simulink model "Quadcopter_Model_Linear"  (R2022a)
settings: Solver=ode45  StartTime=0.0  StopTime=20  RelTol=1e-3
values from neighbouring files (symbols this model uses):
  A = double(subs(a,[x_vec;u],equil))    [A_and_B_Matricies.m]    (also in Controller_LQR.m; Create_System.m; Linear_Main.mat = [0 0 0 0 0 0 0 0 0 0 0 0 ... (81 elements, 9x9)]; Linear_Model.mat = [0 0 0 0 0 0 0 0 0 0 0 1 ... (81 elements, 9x9)])
  B = double(subs(b,[x_vec;u],equil))    [A_and_B_Matricies.m]    (also in Controller_LQR.m; Create_System.m; Linear_Main.mat = [0 0 -1 0 13.2591958939 78.431372549 0 0 0 0 0 -1 ... (36 el; Linear_Model.mat = [0 13.2591958939 0 0 0 0 78.431372549 0 -1 0 0 0 ... (36 ele)
  u_e = zeros(4,1)    [A_and_B_Matricies.m]    (also in Controller_LQR.m; Create_System.m; Linear_Main.mat = [2.45 2.45 2.45 2.45]; Linear_Model.mat = [2.45 2.45 2.45 2.45])
undefined symbols (not defined in the file or in its folder): init, K1, K2, K3, K4
settings Model: Creator=vicen  LastModifiedBy=vicen
settings DebuggingCC: UnconnectedInputMsg=warning  UnconnectedOutputMsg=warning  UnconnectedLineMsg=warning
settings RTWCC: DLArmComputeVersion=19.05

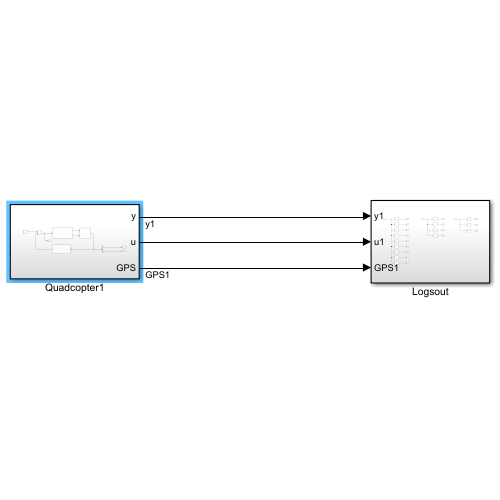
[thumbnail: Simulink's stored preview of the top-level diagram]
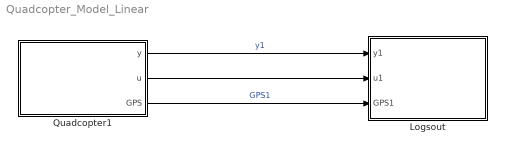
== system Quadcopter_Model_Linear ==
  Logsout : Subsystem
  Quadcopter1 : Subsystem
  wires:
  Quadcopter1/1(y) -> Logsout/1(y1)  "y1"
  Quadcopter1/2(u) -> Logsout/2(u1)
  Quadcopter1/3(GPS) -> Logsout/3(GPS1)  "GPS1"

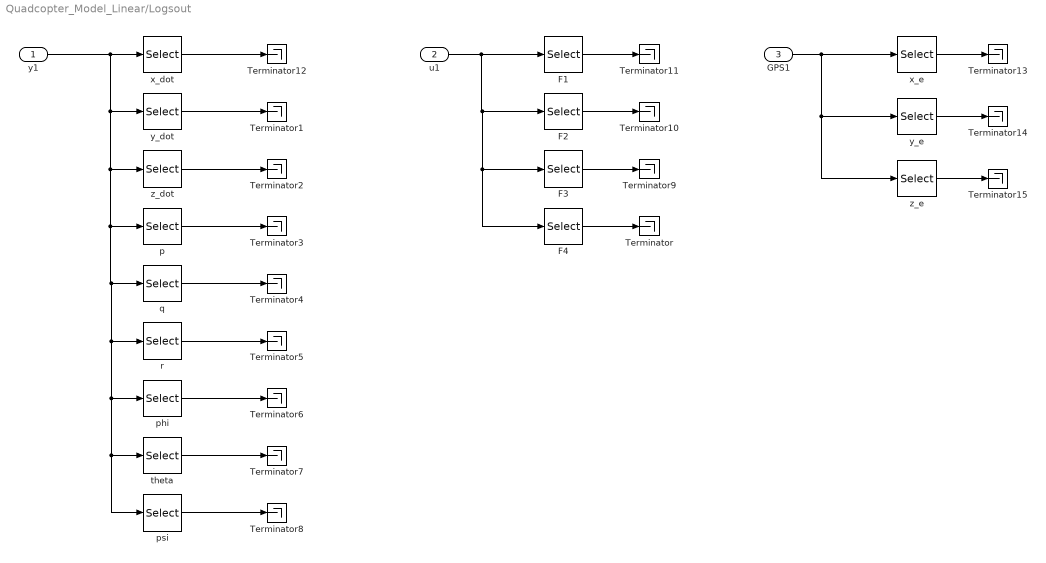
== system Quadcopter_Model_Linear/Logsout ==
  y1 : Inport
  u1 : Inport  Port=2
  GPS1 : Inport  Port=3
  F1 : Selector  InputPortWidth=4  IndexOptions=Index vector (dialog)  Indices=1  OutputSizes=1
  F2 : Selector  InputPortWidth=4  IndexOptions=Index vector (dialog)  Indices=2  OutputSizes=1
  F3 : Selector  InputPortWidth=4  IndexOptions=Index vector (dialog)  Indices=3  OutputSizes=1
  F4 : Selector  InputPortWidth=4  IndexOptions=Index vector (dialog)  Indices=4  OutputSizes=1
  Terminator{,1..15} (16 alike) : Terminator
  p : Selector  InputPortWidth=9  IndexOptions=Index vector (dialog)  Indices=4  OutputSizes=1
  phi : Selector  InputPortWidth=9  IndexOptions=Index vector (dialog)  Indices=7  OutputSizes=1
  psi : Selector  InputPortWidth=9  IndexOptions=Index vector (dialog)  Indices=9  OutputSizes=1
  q : Selector  InputPortWidth=9  IndexOptions=Index vector (dialog)  Indices=5  OutputSizes=1
  r : Selector  InputPortWidth=9  IndexOptions=Index vector (dialog)  Indices=6  OutputSizes=1
  theta : Selector  InputPortWidth=9  IndexOptions=Index vector (dialog)  Indices=8  OutputSizes=1
  x_dot : Selector  InputPortWidth=9  IndexOptions=Index vector (dialog)  Indices=1  OutputSizes=1
  x_e : Selector  InputPortWidth=3  IndexOptions=Index vector (dialog)  Indices=1  OutputSizes=1
  y_dot : Selector  InputPortWidth=9  IndexOptions=Index vector (dialog)  Indices=2  OutputSizes=1
  y_e : Selector  InputPortWidth=3  IndexOptions=Index vector (dialog)  Indices=2  OutputSizes=1
  z_dot : Selector  InputPortWidth=9  IndexOptions=Index vector (dialog)  Indices=3  OutputSizes=1
  z_e : Selector  InputPortWidth=3  IndexOptions=Index vector (dialog)  Indices=3  OutputSizes=1
  wires:
  y1/1 -> psi/1, theta/1, phi/1, r/1, q/1, p/1, z_dot/1, y_dot/1, x_dot/1
  x_dot/1 -> Terminator12/1
  y_dot/1 -> Terminator1/1
  z_dot/1 -> Terminator2/1
  p/1 -> Terminator3/1
  q/1 -> Terminator4/1
  r/1 -> Terminator5/1
  phi/1 -> Terminator6/1
  theta/1 -> Terminator7/1
  psi/1 -> Terminator8/1
  u1/1 -> F4/1, F3/1, F2/1, F1/1
  F1/1 -> Terminator11/1
  F2/1 -> Terminator10/1
  F3/1 -> Terminator9/1
  F4/1 -> Terminator/1
  GPS1/1 -> z_e/1, y_e/1, x_e/1
  x_e/1 -> Terminator13/1
  y_e/1 -> Terminator14/1
  z_e/1 -> Terminator15/1

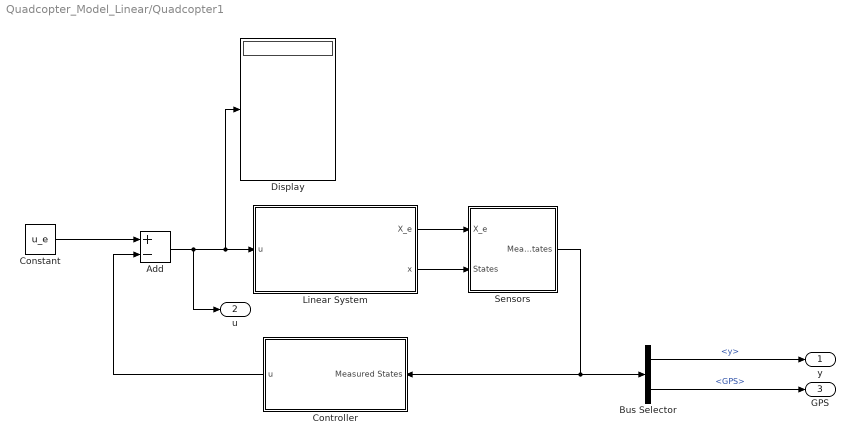
== system Quadcopter_Model_Linear/Quadcopter1 ==
  Add : Sum  Inputs=+-
  Bus Selector : BusSelector  OutputSignals=y,GPS
  Constant : Constant  Value=u_e
  Controller : Subsystem
  Display : Display
  Linear System : Subsystem
  Sensors : Subsystem
  y : Outport
  u : Outport  Port=2
  GPS : Outport  Port=3
  wires:
  Linear System/1(X_e) -> Sensors/1(X_e)
  Linear System/2(x) -> Sensors/2(States)
  Sensors/1(Measured States) -> Controller/1(Measured States), Bus Selector/1
  Bus Selector/2 -> GPS/1  "<GPS>"
  Bus Selector/1 -> y/1  "<y>"
  Controller/1(u) -> Add/2
  Add/1 -> u/1, Display/1, Linear System/1(u)
  Constant/1 -> Add/1

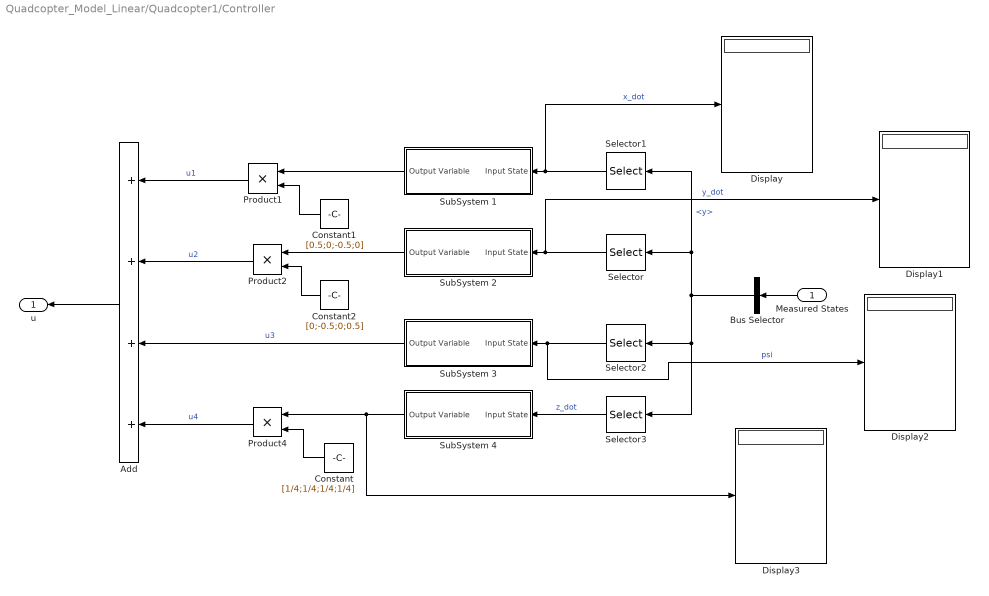
== system Quadcopter_Model_Linear/Quadcopter1/Controller ==
  Measured States : Inport
  Add : Sum  Inputs=++++
  Bus Selector : BusSelector  OutputSignals=y
  Constant : Constant  Value=[1/4;1/4;1/4;1/4]
  Constant1 : Constant  Value=[0.5;0;-0.5;0]
  Constant2 : Constant  Value=[0;-0.5;0;0.5]
  Display{,1..3} (4 alike) : Display
  Product1 : Product
  Product2 : Product
  Product4 : Product
  Selector : Selector  InputPortWidth=9  IndexOptions=Index vector (dialog)  Indices=2  OutputSizes=1
  Selector1 : Selector  InputPortWidth=9  IndexOptions=Index vector (dialog)  Indices=1  OutputSizes=1
  Selector2 : Selector  InputPortWidth=9  IndexOptions=Index vector (dialog)  Indices=[6 9]  OutputSizes=1
  Selector3 : Selector  InputPortWidth=9  IndexOptions=Index vector (dialog)  Indices=3  OutputSizes=1
  SubSystem 1 : Subsystem
  SubSystem 2 : Subsystem
  SubSystem 3 : Subsystem
  SubSystem 4 : Subsystem
  u : Outport
  wires:
  Add/1 -> u/1
  Product1/1 -> Add/1  "u1"
  SubSystem 3/1(Output Variable) -> Add/3  "u3"
  Product4/1 -> Add/4  "u4"
  Measured States/1 -> Bus Selector/1
  Bus Selector/1 -> Selector1/1, Selector/1, Selector3/1, Selector2/1  "<y>"
  Selector1/1 -> Display/1, SubSystem 1/1(Input State)  "x_dot"
  Selector/1 -> Display1/1, SubSystem 2/1(Input State)  "y_dot"
  Selector2/1 -> Display2/1, SubSystem 3/1(Input State)  "psi"
  Selector3/1 -> SubSystem 4/1(Input State)  "z_dot"
  SubSystem 4/1(Output Variable) -> Display3/1, Product4/1
  Constant/1 -> Product4/2
  Constant1/1 -> Product1/2
  Constant2/1 -> Product2/2
  Product2/1 -> Add/2  "u2"
  SubSystem 1/1(Output Variable) -> Product1/1
  SubSystem 2/1(Output Variable) -> Product2/1

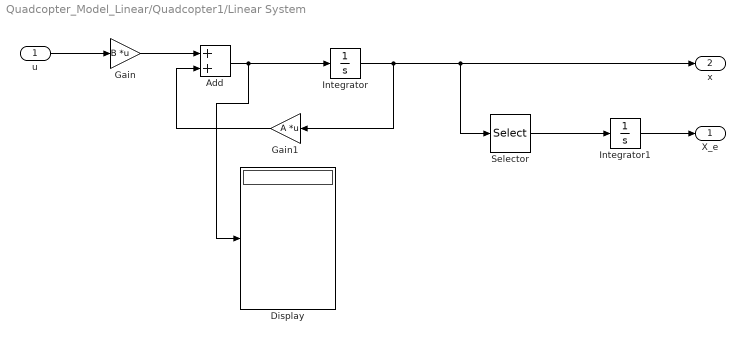
== system Quadcopter_Model_Linear/Quadcopter1/Linear System ==
  u : Inport
  Add : Sum
  Display : Display
  Gain : Gain  Gain=B  Multiplication=Matrix(K*u)
  Gain1 : Gain  Gain=A  Multiplication=Matrix(K*u)
  Integrator : Integrator  InitialCondition=[init.vel_b';init.rotation_rates_b';init.Euler']
  Integrator1 : Integrator  InitialCondition=init.pos_e'
  Selector : Selector  InputPortWidth=9  IndexOptions=Index vector (dialog)  Indices=[1 2 3]  OutputSizes=1
  X_e : Outport
  x : Outport  Port=2
  wires:
  u/1 -> Gain/1
  Gain/1 -> Add/1
  Add/1 -> Display/1, Integrator/1
  Integrator/1 -> x/1, Selector/1, Gain1/1
  Gain1/1 -> Add/2
  Selector/1 -> Integrator1/1
  Integrator1/1 -> X_e/1

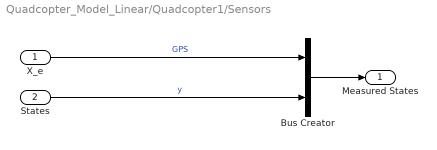
== system Quadcopter_Model_Linear/Quadcopter1/Sensors ==
  X_e : Inport
  States : Inport  Port=2
  Bus Creator : BusCreator  Inputs=2
  Measured States : Outport
  wires:
  States/1 -> Bus Creator/2  "y"
  Bus Creator/1 -> Measured States/1
  X_e/1 -> Bus Creator/1  "GPS"

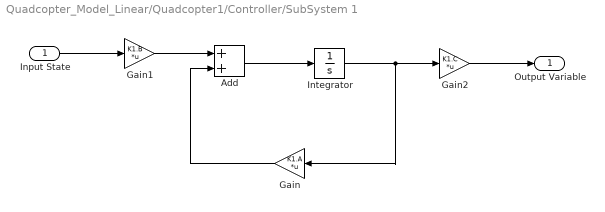
== system Quadcopter_Model_Linear/Quadcopter1/Controller/SubSystem 1 ==
  Input State : Inport
  Add : Sum
  Gain : Gain  Gain=K1.A  Multiplication=Matrix(K*u)
  Gain1 : Gain  Gain=K1.B  Multiplication=Matrix(K*u)
  Gain2 : Gain  Gain=K1.C  Multiplication=Matrix(K*u)
  Integrator : Integrator
  Output Variable : Outport
  wires:
  Input State/1 -> Gain1/1
  Gain1/1 -> Add/1
  Add/1 -> Integrator/1
  Integrator/1 -> Gain2/1, Gain/1
  Gain/1 -> Add/2
  Gain2/1 -> Output Variable/1

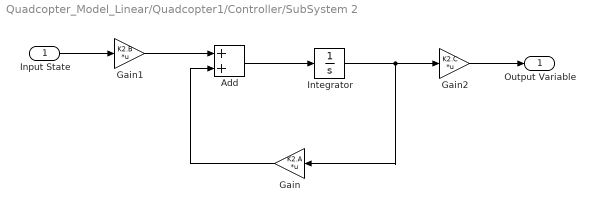
== system Quadcopter_Model_Linear/Quadcopter1/Controller/SubSystem 2 ==
  Input State : Inport
  Add : Sum
  Gain : Gain  Gain=K2.A  Multiplication=Matrix(K*u)
  Gain1 : Gain  Gain=K2.B  Multiplication=Matrix(K*u)
  Gain2 : Gain  Gain=K2.C  Multiplication=Matrix(K*u)
  Integrator : Integrator
  Output Variable : Outport
  wires:
  Gain/1 -> Add/2
  Integrator/1 -> Gain/1, Gain2/1
  Add/1 -> Integrator/1
  Gain1/1 -> Add/1
  Input State/1 -> Gain1/1
  Gain2/1 -> Output Variable/1

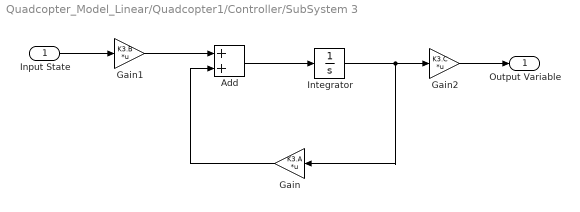
== system Quadcopter_Model_Linear/Quadcopter1/Controller/SubSystem 3 ==
  Input State : Inport
  Add : Sum
  Gain : Gain  Gain=K3.A  Multiplication=Matrix(K*u)
  Gain1 : Gain  Gain=K3.B  Multiplication=Matrix(K*u)
  Gain2 : Gain  Gain=K3.C  Multiplication=Matrix(K*u)
  Integrator : Integrator
  Output Variable : Outport
  wires:
  Input State/1 -> Gain1/1
  Gain1/1 -> Add/1
  Add/1 -> Integrator/1
  Integrator/1 -> Gain2/1, Gain/1
  Gain/1 -> Add/2
  Gain2/1 -> Output Variable/1

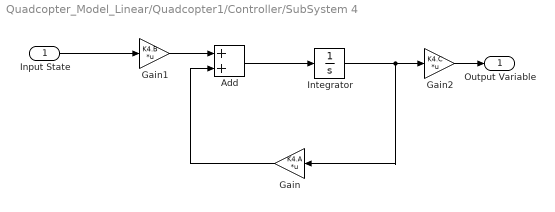
== system Quadcopter_Model_Linear/Quadcopter1/Controller/SubSystem 4 ==
  Input State : Inport
  Add : Sum
  Gain : Gain  Gain=K4.A  Multiplication=Matrix(K*u)
  Gain1 : Gain  Gain=K4.B  Multiplication=Matrix(K*u)
  Gain2 : Gain  Gain=K4.C  Multiplication=Matrix(K*u)
  Integrator : Integrator
  Output Variable : Outport
  wires:
  Gain/1 -> Add/2
  Integrator/1 -> Gain/1, Gain2/1
  Add/1 -> Integrator/1
  Gain1/1 -> Add/1
  Input State/1 -> Gain1/1
  Gain2/1 -> Output Variable/1
